simulink model "vana_yeni_model_harness"  (R2025b)
settings: Solver=FixedStepAuto  StartTime=0.0  StopTime=23  FixedStep=1e-3  RelTol=1e-3
values from neighbouring files (symbols this model uses):
  SimCoef = [flipud(Plant_Coef); 0]'    [vana_yeni_model_matlab.m]
settings Model: Creator=Kaan Kalkandelen  LastModifiedBy=Kaan Kalkandelen

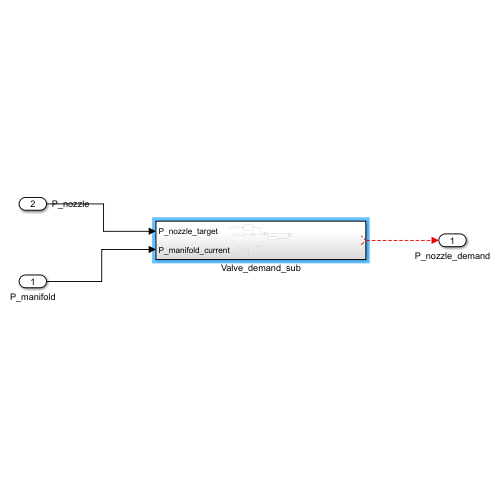
[thumbnail: Simulink's stored preview of the top-level diagram]
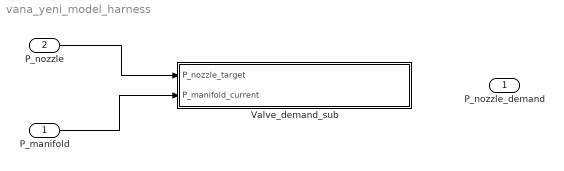
== system vana_yeni_model_harness ==
  P_manifold : Inport
  P_nozzle : Inport  Port=2
  Valve_demand_sub : Subsystem
  P_nozzle_demand : Outport
  wires:
  P_manifold/1 -> Valve_demand_sub/2(P_manifold_current)
  P_nozzle/1 -> Valve_demand_sub/1(P_nozzle_target)
  ? -> P_nozzle_demand/1

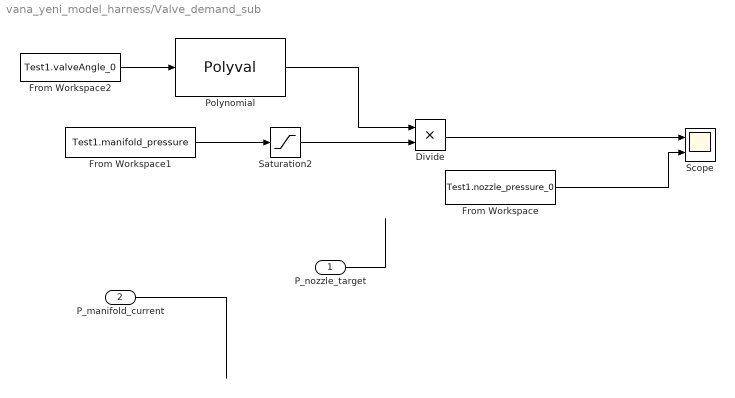
== system vana_yeni_model_harness/Valve_demand_sub ==
  P_nozzle_target : Inport
  P_manifold_current : Inport  Port=2
  Divide : Product  Inputs=**
  From Workspace : FromWorkspace  VariableName=Test1.nozzle_pressure_0  OutputAfterFinalValue=Setting to zero
  From Workspace1 : FromWorkspace  VariableName=Test1.manifold_pressure
  From Workspace2 : FromWorkspace  VariableName=Test1.valveAngle_0  OutputAfterFinalValue=Setting to zero
  Polynomial : Polyval  Coefs=SimCoef
  Saturation2 : Saturate  UpperLimit=inf  LowerLimit=14
  Scope : Scope  NumInputPorts=2
      settings: ActiveDisplayYMinimum=-165.00308693998349  ActiveDisplayYMaximum=1227.5554422771852
  wires:
  P_manifold_current/1 -> ?
  P_nozzle_target/1 -> ?
  From Workspace/1 -> Scope/2
  From Workspace1/1 -> Saturation2/1
  From Workspace2/1 -> Polynomial/1
  Divide/1 -> Scope/1
  Polynomial/1 -> Divide/1
  Saturation2/1 -> Divide/2
